simulink model "pengukuran_dasar"  (R2025a)
settings: Solver=VariableStepAuto  StartTime=0.0  StopTime=10.0  RelTol=1e-3
libraries: spsSeriesRLCBranchLib x10, spsDCVoltageSourceLib x6, sps_lib x6, spsCurrentMeasurementLib x4, spsVoltageMeasurementLib x4
settings Model: Creator=pasha  LastModifiedBy=pasha

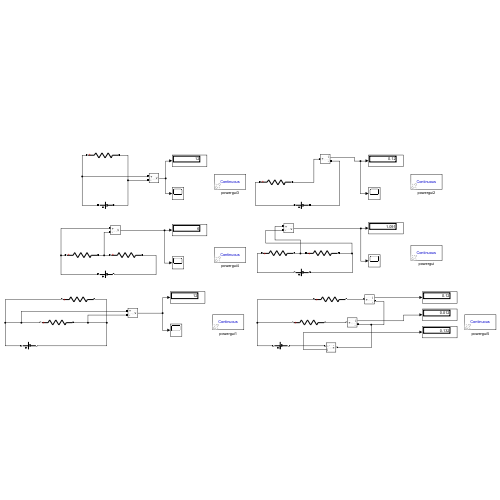
[thumbnail: Simulink's stored preview of the top-level diagram]
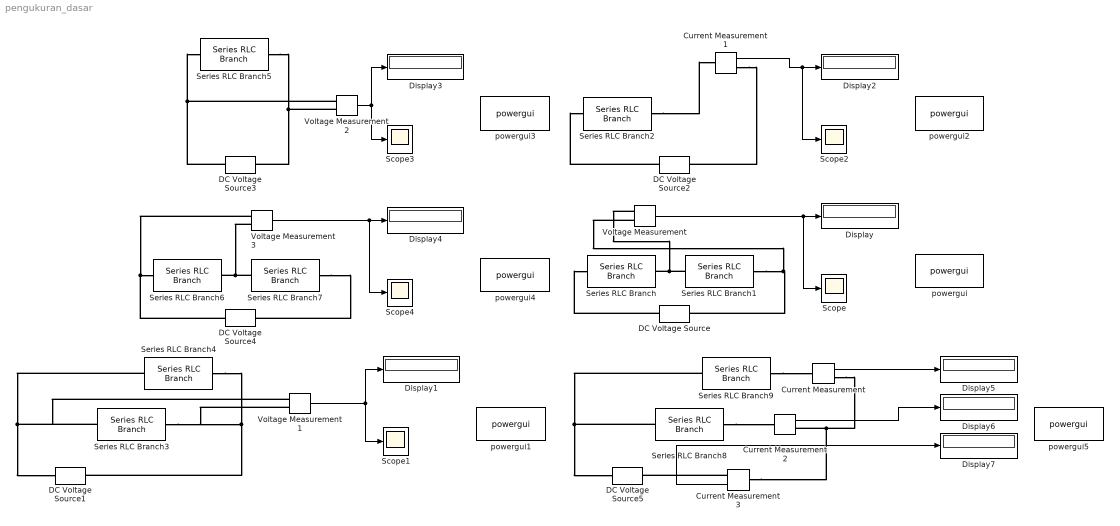
== system pengukuran_dasar ==
  Current Measurement{,1..3} (4 alike) : spsCurrentMeasurementLib/Current Measurement  PhasorSimulation=off  OutputType=Complex  PSBequivalent=0
  DC Voltage Source{,1..5} (6 alike) : spsDCVoltageSourceLib/DC Voltage Source  Amplitude=12  Measurements=None
  Display{,1..7} (8 alike) : Display
  Scope{,1..4} (5 alike) : Scope
      Scope settings: ActiveDisplayYMinimum=-1  ActiveDisplayYMaximum=1
      Scope1 settings: ActiveDisplayYMinimum=-1  ActiveDisplayYMaximum=1
      Scope2 settings: ActiveDisplayYMinimum=-1  ActiveDisplayYMaximum=1  DataLoggingVariableName=ScopeData2
      Scope3 settings: ActiveDisplayYMinimum=-1  ActiveDisplayYMaximum=1  DataLoggingVariableName=ScopeData3
      Scope4 settings: ActiveDisplayYMinimum=-1  ActiveDisplayYMaximum=1  DataLoggingVariableName=ScopeData4
  Series RLC Branch{,3..4,6..8} (6 alike) : spsSeriesRLCBranchLib/Series RLC Branch  LConnTagsString=__new0  RConnTagsString=__new0  BranchType=R  Resistance=1000  Inductance=1e-3  SetiL0=off  InitialCurrent=0  Capacitance=1e-6  Setx0=off  InitialVoltage=0  Measurements=None
  Series RLC Branch{1..2,5,9} (4 alike) : spsSeriesRLCBranchLib/Series RLC Branch  LConnTagsString=__new0  RConnTagsString=__new0  BranchType=R  Resistance=100  Inductance=1e-3  SetiL0=off  InitialCurrent=0  Capacitance=1e-6  Setx0=off  InitialVoltage=0  Measurements=None
  Voltage Measurement{,1..3} (4 alike) : spsVoltageMeasurementLib/Voltage Measurement  PhasorSimulation=off  OutputType=Complex  PSBequivalent=0
  powergui{,1..5} (6 alike) : sps_lib/powergui  Priority=1  SimulationMode=Continuous  SampleTime=50e-6  frequency=60  Iterations=50  frequencyindice=0  Pbase=100e6  ErrMax=1e-4  UnitsV=kV  UnitsW=MW  buscounter=0  FunctionMessages=off  echomessages=off  EnableUseOfTLC=off  CurrentSourceSwitches=off  DisableSnubberDevices=off  DisableRonSwitches=off  DisableVfSwitches=off  DisplayEquations=off  AutomaticDiscreteSolvers=off  SolverType=Tustin/Backward Euler (TBE)  Interpol=off  ExternalGateDelay=off  methode=off  Ts=100  x0status=blocks  SPID=on  SwTol=0  HookPort=off  NonlinearTolerance=1e-4  nMaxIteration=100  ContinueOnMaxIteration=off  RestoreLinks=warning  ResistiveCurrentMeasurement=off  Frange=[0:2:500]  Ylog=off  Xlog=on  ShowGrid=off  save=off  variable=ZData  structure=0  ZoomFFT=off  StartTime=0.0  cycles=1  DisplayStyle=1  fundamental=60  FreqAxis=off  MaxFrequency=1000  frequencyindicesteady=1  RmsSteady=1  display=off
  wires:
  Voltage Measurement/1 -> Display/1, Scope/1
  Current Measurement1/1 -> Scope2/1, Display2/1
  Voltage Measurement1/1 -> Display1/1, Scope1/1
  Voltage Measurement2/1 -> Display3/1, Scope3/1
  Voltage Measurement3/1 -> Display4/1, Scope4/1
  Current Measurement/1 -> Display5/1
  Current Measurement2/1 -> Display6/1
  Current Measurement3/1 -> Display7/1
  connections:
  DC Voltage Source/RConn1 -- Series RLC Branch/LConn1
  Series RLC Branch1/LConn1 -- Voltage Measurement/LConn1 -- Series RLC Branch/RConn1
  Series RLC Branch1/RConn1 -- Voltage Measurement/LConn2 -- DC Voltage Source/LConn1
  Series RLC Branch2/RConn1 -- Current Measurement1/LConn1
  Current Measurement1/RConn1 -- DC Voltage Source2/LConn1
  DC Voltage Source2/RConn1 -- Series RLC Branch2/LConn1
  Series RLC Branch4/LConn1 -- Voltage Measurement1/LConn1 -- Series RLC Branch3/LConn1 -- DC Voltage Source1/RConn1
  Series RLC Branch4/RConn1 -- Series RLC Branch3/RConn1 -- Voltage Measurement1/LConn2 -- DC Voltage Source1/LConn1
  DC Voltage Source3/RConn1 -- Voltage Measurement2/LConn1 -- Series RLC Branch5/LConn1
  Series RLC Branch5/RConn1 -- Voltage Measurement2/LConn2 -- DC Voltage Source3/LConn1
  Series RLC Branch7/LConn1 -- Voltage Measurement3/LConn2 -- Series RLC Branch6/RConn1
  Series RLC Branch7/RConn1 -- DC Voltage Source4/LConn1
  DC Voltage Source4/RConn1 -- Voltage Measurement3/LConn1 -- Series RLC Branch6/LConn1
  Series RLC Branch8/LConn1 -- DC Voltage Source5/RConn1 -- Series RLC Branch9/LConn1
  Series RLC Branch9/RConn1 -- Current Measurement/LConn1
  Series RLC Branch8/RConn1 -- Current Measurement2/LConn1
  Current Measurement/RConn1 -- Current Measurement3/LConn1 -- Current Measurement2/RConn1
  Current Measurement3/RConn1 -- DC Voltage Source5/LConn1
